simulink model "filterTest"  (R2015a)
settings: Solver=ode45  StartTime=0.0  StopTime=10.0  RelTol=1e-3
libraries: dsparch4 x1
settings Model: Creator=John  LastModifiedBy=John

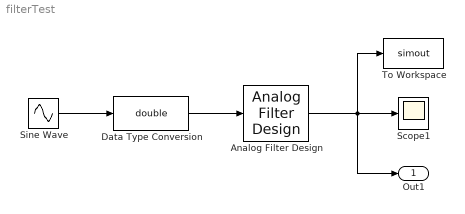
== system filterTest ==
  Analog Filter Design : dsparch4/Analog Filter Design  method=Butterworth  filttype=Lowpass  N=8  Wlo=30  Whi=80  Rp=2  Rs=40
  Data Type Conversion : DataTypeConversion  OutDataTypeStr=double
  Scope1 : Scope
  Sine Wave : Sin  SampleTime=0
  To Workspace : ToWorkspace  VariableName=simout  SaveFormat=Timeseries  SampleTime=-1
  Out1 : Outport
  wires:
  Analog Filter Design/1 -> Out1/1, To Workspace/1, Scope1/1
  Sine Wave/1 -> Data Type Conversion/1
  Data Type Conversion/1 -> Analog Filter Design/1
